simulink model "asserv_etat_lqr_hil_r2019b"  (R2019b)
settings: Solver=FixedStepAuto  StartTime=0.0  StopTime=inf  FixedStep=0.002  RelTol=1e-3  EnableMultiTasking=on
PostLoadFcn:
  | qc_set_target_type(getConfigSet(bdroot, 'QUARC Default Target Configuration'));
values from neighbouring files (symbols this model uses):
  g = 0.01    [asserv_etat_etendu_ini.m]    (also in identification_ini.m = 0.008703; identification_opt.m = x(4))
  Kt = 0.5    [asserv_etat_etendu_ini.m]    (also in identification_ini.m; identification_opt.m)
  Kv = 35.0    (= 35)    [asserv_etat_etendu_ini.m]    (also in identification_ini.m = 45.608692; identification_opt.m = x(1))
  L = [L(2) L(1) L(3)]    [asserv_etat_etendu_ini.m]    (also in asserv_etat_ini.m = [1 0]; asserv_etat_lqr_ini.m)
  tau_e = 0.003    [asserv_etat_etendu_ini.m]    (also in identification_ini.m = 0.002853; identification_opt.m = x(3))
  tau_m = 0.015    [asserv_etat_etendu_ini.m]    (also in identification_ini.m = 0.015641; identification_opt.m = x(2))
  Te = 0.002    [asserv_avance_phase_ini.m]    (also in asserv_etat_etendu_ini.m; identification_ini.m; identification_opt.m)
undefined symbols (not defined in the file or in its folder): HIL
libraries: quarc_library x5
Description:
  | This example is a simple analog loopback test. It sends a signal to analog output
  | channel #0 and then reads analog input channel #0. Wire analog output #0 to analog
  | input #0 to see the signal on the Scope. Change the amplitude of the signal and see
  | the change occur on the Scope.
settings Model: SimulationMode=external  ExtModeTrigDuration=10000  Creator=drmadill  LastModifiedBy=collette
settings SolverCC: PositivePriorityOrder=on
settings DataIOCC: LimitDataPoints=on  SaveFormat=Array  SignalLoggingSaveFormat=ModelDataLogs  ReturnWorkspaceOutputs=off
settings OptimizationCC: ExpressionDepthLimit=2147483647  InitFltsAndDblsToZero=on  LifeSpan=inf
settings DebuggingCC: SaveWithParameterizedLinksMsg=none  UnderspecifiedInitializationDetection=Classic  MergeDetectMultiDrivingBlocksExec=none  SolverPrmCheckMsg=warning  FcnCallInpInsideContextMsg=warning  StateNameClashWarn=warning  SFUnexpectedBacktrackingDiag=warning  SFNoUnconditionalDefaultTransitionDiag=warning  ArithmeticOperatorsInVariantConditions=warning
settings HardwareCC: ProdBitPerPointer=32  ProdBitPerSizeT=32  ProdBitPerPtrDiffT=32  ProdLargestAtomicFloat=None  ProdIntDivRoundTo=Undefined  ProdEndianess=Unspecified  ProdWordSize=32  ProdHWDeviceType=32-bit Generic
settings ModelReferenceCC: PropagateSignalLabelsOutOfModel=off
settings SFSimCC: SimUseLocalCustomCode=off  CustomCodeUndefinedFunction=UseInterfaceOnly
settings RTWCC: Description=QUARC Win64 Target  SystemTargetFile=quarc_win64.tlc  TemplateMakefile=quarc_default_tmf  RTWUseLocalCustomCode=off
settings CodeAppCC: StateflowObjectComments=on
settings STFCustomTargetCC: TargetPreCompLibLocation=C:\PROGRA~3\QUARC\lib\2020a\win64\release  ConcurrentExecutionCompliant=on  CPPClassGenCompliant=on  GRTInterface=on  SystemTargetFile=quarc_win64.tlc
settings GRTTargetCC: TargetPreCompLibLocation=C:\PROGRA~3\QUARC\lib\2020a\win64\release  TargetLangStandard=C89/C90 (ANSI)  ParMdlRefBuildCompliant=off  CompOptLevelCompliant=off  CombineOutputUpdateFcns=off  MatFileLogging=off  GRTInterface=on  UseToolchainInfoCompliant=off  ExtMode=on  ExtModeMexFile=quarc_comm
settings ConfigComp: CovMetricSettings=dw  CovHtmlReporting=on  CovSaveCumulativeToWorkspaceVar=on  CovSaveSingleToWorkspaceVar=on  CovExternalEMLEnable=off

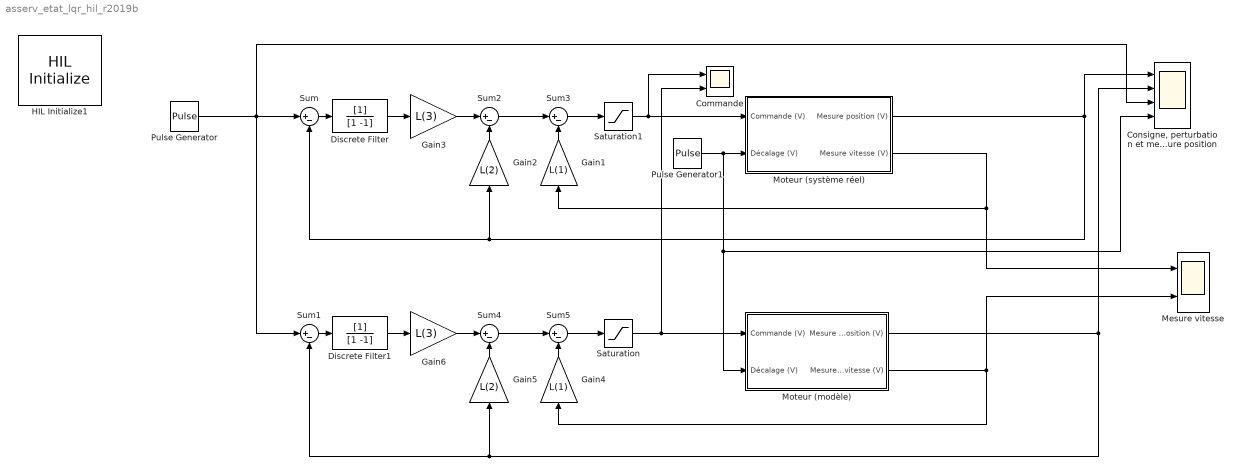
== system asserv_etat_lqr_hil_r2019b ==
  Commande : Scope  NumInputPorts=2
  "Consigne, perturbation et mesure position" : Scope  NumInputPorts=4
  Discrete Filter : DiscreteFilter  Denominator=[1 -1]  SampleTime=Te
  Discrete Filter1 : DiscreteFilter  Denominator=[1 -1]  SampleTime=Te
  Gain1 : Gain  Gain=L(1)
  Gain2 : Gain  Gain=L(2)
  Gain3 : Gain  Gain=L(3)
  Gain4 : Gain  Gain=L(1)
  Gain5 : Gain  Gain=L(2)
  Gain6 : Gain  Gain=L(3)
  HIL Initialize1 : quarc_library/Data Acquisition/Generic/Configuration/HIL Initialize  object_name=HIL-1  board_type=q2_usb  board_number=0  board_options=d0=digital;d1=digital;led=auto;update_rate=fast;decimation=1  exclusive=off  active=on  hardware_clocks=[0]  clock_modes=[]  initial_clock_frequencies=[]  set_clock_params_at_start=off  set_clock_params_at_switch_in=off  set_clock_frequencies_at_start=off  set_clock_frequencies_at_switch_in=off  analog_input_channels=[0:1]  analog_input_configurations=[]  analog_input_maximums=10  analog_input_minimums=-10  set_analog_input_params_at_start=on  set_analog_input_params_at_switch_in=off  analog_output_channels=[0:1]  analog_output_maximums=10  analog_output_minimums=-10  initial_analog_outputs=[0]  final_analog_outputs=[0]  watchdog_analog_outputs=0  set_analog_output_params_at_start=on  set_analog_output_params_at_switch_in=off  set_analog_outputs_at_start=on  set_analog_outputs_at_switch_in=off  set_analog_outputs_at_terminate=on  set_analog_outputs_at_switch_out=off  set_analog_outputs_on_watchdog=off  digital_input_channels=[]  digital_output_channels=[]  digital_output_configuration=[]  initial_digital_outputs=[1]  final_digital_outputs=[1]  watchdog_digital_outputs=[1]  set_digital_output_params_at_start=off  set_digital_output_params_at_switch_in=off  set_digital_outputs_at_start=on  set_digital_outputs_at_switch_in=off  set_digital_outputs_at_terminate=on  set_digital_outputs_at_switch_out=off  set_digital_outputs_on_watchdog=off  encoder_channels=[0:1]  quadrature=[4]  encoder_filter_frequency=[]  initial_encoder_counts=[0]  set_encoder_params_at_start=on  set_encoder_params_at_switch_in=off  set_encoder_counts_at_start=on  set_encoder_counts_at_switch_in=off  pwm_channels=[]  pwm_modes=[0]  pwm_frequency=1/0.020  pwm_configuration=[]  pwm_alignment=[]  pwm_polarity=[]  pwm_leading_deadband=[]  pwm_trailing_deadband=[]  initial_pwm_outputs=[0]  final_pwm_outputs=[0]  watchdog_pwm_outputs=[0]  set_pwm_params_at_start=on  set_pwm_params_at_switch_in=off  set_pwm_outputs_at_start=on  set_pwm_outputs_at_switch_in=off  set_pwm_outputs_at_terminate=on  set_pwm_outputs_at_switch_out=off  set_pwm_outputs_on_watchdog=off  other_output_channels=[]  initial_other_outputs=[]  final_other_outputs=[]  watchdog_other_outputs=[]  set_other_outputs_at_start=off  set_other_outputs_at_switch_in=off  set_other_outputs_at_terminate=off  set_other_outputs_at_switch_out=off  set_other_outputs_on_watchdog=off
  Mesure vitesse : Scope  NumInputPorts=2
  Moteur (modèle) : Subsystem  mask{Parameter1=Kv, Parameter2=Kt, Parameter3=g, Parameter4=tau_m, Parameter5=tau_e, Parameter6=Te}
      mask prompts: Parameter1 "Kv"; Parameter2 "Kt"; Parameter3 "g"; Parameter4 "tau_m"; Parameter5 "tau_e"; Parameter6 "Te"
  Moteur (système réel) : Subsystem
  Pulse Generator : DiscretePulseGenerator  PulseType=Time based  Amplitude=2  PulseWidth=50
  Pulse Generator1 : DiscretePulseGenerator  PulseType=Time based  Amplitude=4  PulseWidth=50  PhaseDelay=0.5
  Saturation : Saturate  UpperLimit=10  LowerLimit=-10
  Saturation1 : Saturate  UpperLimit=10  LowerLimit=-10
  Sum{,1..5} (6 alike) : Sum  Inputs=|+-
  wires:
  Discrete Filter/1 -> Gain3/1
  Gain2/1 -> Sum2/2
  Pulse Generator1/1 -> Moteur (système réel)/2(Décalage (V)), "Consigne, perturbation et mesure position"/4, Moteur (modèle)/2(Décalage (V))
  Moteur (système réel)/1(Mesure position (V)) -> Sum/2, Gain2/1, "Consigne, perturbation et mesure position"/1
  Pulse Generator/1 -> Sum1/1, "Consigne, perturbation et mesure position"/3, Sum/1
  Gain3/1 -> Sum2/1
  Moteur (système réel)/2(Mesure vitesse (V)) -> Gain1/1, Mesure vitesse/1
  Sum/1 -> Discrete Filter/1
  Sum2/1 -> Sum3/1
  Sum3/1 -> Saturation1/1
  Gain1/1 -> Sum3/2
  Gain4/1 -> Sum5/2
  Sum4/1 -> Sum5/1
  Sum5/1 -> Saturation/1
  Sum1/1 -> Discrete Filter1/1
  Gain5/1 -> Sum4/2
  Discrete Filter1/1 -> Gain6/1
  Gain6/1 -> Sum4/1
  Saturation/1 -> Commande/2, Moteur (modèle)/1(Commande (V))
  Saturation1/1 -> Commande/1, Moteur (système réel)/1(Commande (V))
  Moteur (modèle)/1(Mesure position (V)) -> "Consigne, perturbation et mesure position"/2, Sum1/2, Gain5/1
  Moteur (modèle)/2(Mesure vitesse (V)) -> Gain4/1, Mesure vitesse/2

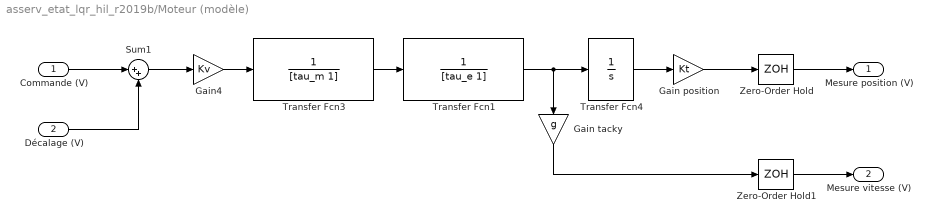
== system asserv_etat_lqr_hil_r2019b/Moteur (modèle) ==
  Commande (V) : Inport
  Décalage (V) : Inport  Port=2
  Gain position : Gain  Gain=Kt
  Gain tacky : Gain  Gain=g
  Gain4 : Gain  Gain=Kv
  Sum1 : Sum  Inputs=|++
  Transfer Fcn1 : TransferFcn  Denominator=[tau_e 1]
  Transfer Fcn3 : TransferFcn  Denominator=[tau_m 1]
  Transfer Fcn4 : TransferFcn  Denominator=[1 0]
  Zero-Order Hold : ZeroOrderHold  SampleTime=Te
  Zero-Order Hold1 : ZeroOrderHold  SampleTime=Te
  Mesure position (V) : Outport
  Mesure vitesse (V) : Outport  Port=2
  wires:
  Gain tacky/1 -> Zero-Order Hold1/1
  Transfer Fcn3/1 -> Transfer Fcn1/1
  Transfer Fcn4/1 -> Gain position/1
  Gain position/1 -> Zero-Order Hold/1
  Gain4/1 -> Transfer Fcn3/1
  Commande (V)/1 -> Sum1/1
  Sum1/1 -> Gain4/1
  Décalage (V)/1 -> Sum1/2
  Transfer Fcn1/1 -> Transfer Fcn4/1, Gain tacky/1
  Zero-Order Hold/1 -> Mesure position (V)/1
  Zero-Order Hold1/1 -> Mesure vitesse (V)/1

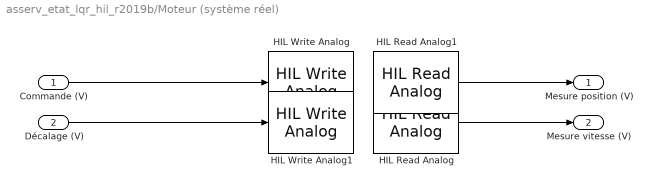
== system asserv_etat_lqr_hil_r2019b/Moteur (système réel) ==
  Commande (V) : Inport
  Décalage (V) : Inport  Port=2
  HIL Read Analog : quarc_library/Data Acquisition/Generic/Immediate I//O/HIL Read Analog  Tag=unassigned  object_name=HIL-1  channels=1  sample_time=qc_get_step_size  active=on  vector_output=off
  HIL Read Analog1 : quarc_library/Data Acquisition/Generic/Immediate I//O/HIL Read Analog  Tag=unassigned  object_name=HIL-1  channels=0  sample_time=qc_get_step_size  active=on  vector_output=off
  HIL Write Analog : quarc_library/Data Acquisition/Generic/Immediate I//O/HIL Write Analog  Tag=unassigned  object_name=HIL-1  channels=0  sample_time=-1  active=on  vector_input=off
  HIL Write Analog1 : quarc_library/Data Acquisition/Generic/Immediate I//O/HIL Write Analog  Tag=unassigned  object_name=HIL-1  channels=1  sample_time=-1  active=on  vector_input=off
  Mesure position (V) : Outport
  Mesure vitesse (V) : Outport  Port=2
  wires:
  Décalage (V)/1 -> HIL Write Analog1/1
  Commande (V)/1 -> HIL Write Analog/1
  HIL Read Analog1/1 -> Mesure position (V)/1
  HIL Read Analog/1 -> Mesure vitesse (V)/1
